simulink model "ThdRwRtStBkReclnIsPosChk"  (R2018b)
settings: Solver=FixedStepDiscrete  StartTime=0.0  StopTime=10.0  FixedStep=0.01  RelTol=1e-3
undefined symbols (not defined in the file or in its folder): KeSMSuThrdRwStBackPosDelta_Val, KeSMSuThrdRwStBackPosTolr_Val, KeSMSuVehicleModelConfig_Val
libraries: StIsPosChkLib x12, simulink x5
settings Model: Creator=sn2xws  LastModifiedBy=sn55gm
settings Model: ModifiedHistory=|
  | 2024.3.14
  | V2.3.0
  | Bug 813950 童锁Lock，Mode1_Easy Entry Mode 不应调用失败
  | 2024.6.25
  | V3.0.0 557模式流程
  | 2024.9.6 V3.0.1 新增Md56
  | 2024.10.14 V3.0.2 新增Md57，Md58
  | 2024.11.11 V3.0.3 vip模式到位置不看三排
  | 2024.11.27.V3.0.4 Md57 Md58接线遗漏
  | 2025.2.19 V3.8.0 Bug 991386 Md1 三排占座时未移动且报了成功
  | 25.7.1 V3.13.0 新增MD61 MD62
settings DataIOCC: SaveFormat=StructureWithTime
settings OptimizationCC: DefaultParameterBehavior=Inlined  EnhancedBackFolding=on  PassReuseOutputArgsAs=Individual arguments  ZeroExternalMemoryAtStartup=off  ZeroInternalMemoryAtStartup=off  OptimizeBlockOrder=speed  DifferentSizesBufferReuse=on  OptimizationCustomize=off
settings DebuggingCC: ParameterTunabilityLossMsg=error
settings ModelReferenceCC: ModelReferenceNumInstancesAllowed=Single
settings SFSimCC: MATLABDynamicMemAlloc=off
settings RTWCC: SystemTargetFile=autosar.tlc  GenCodeOnly=on  TemplateMakefile=ert_default_tmf  Description=AUTOSAR  GenerateReport=on  IncludeHyperlinkInReport=on  LaunchReport=on  GenerateTraceInfo=on  GenerateTraceReport=on  GenerateTraceReportSl=on  GenerateTraceReportSf=on  GenerateTraceReportEml=on
settings CodeAppCC: ForceParamTrailComments=on  IgnoreCustomStorageClasses=off  OperatorAnnotations=on  SimulinkDataObjDesc=on  SFDataObjDesc=on  InsertBlockDesc=on
settings STFCustomTargetCC: TargetLangStandard=C99 (ISO)  MultiwordLength=256  ParMdlRefBuildCompliant=on  CompOptLevelCompliant=on  IncludeMdlTerminateFcn=off  CombineOutputUpdateFcns=on  SuppressErrorStatus=on  ERTCustomFileBanners=on  SupportNonFinite=off  SupportComplex=off  SupportContinuousTime=off  SupportNonInlinedSFcns=off  RemoveResetFunc=on  MATLABClassNameForMDSCustomization=Simulink.SoftwareTarget.ERTCustomization  AutosarCompliant=on  UseToolchainInfoCompliant=on  LookupTableObjectStructAxisOrder=2,1,3,4,...  LUTObjectStructOrderEvenSpacing=Size,Table,Breakpoints  SystemTargetFile=autosar.tlc
settings ERTTargetCC: TargetLangStandard=C99 (ISO)  ConcurrentExecutionCompliant=off  IncludeMdlTerminateFcn=off  SuppressErrorStatus=on  SupportNonFinite=off  SupportComplex=off  ModelStepFunctionPrototypeControlCompliant=off  CPPClassGenCompliant=off  AutosarCompliant=on  LookupTableObjectStructAxisOrder=2,1,3,4,...  LUTObjectStructOrderEvenSpacing=Size,Table,Breakpoints  InlinedParameterPlacement=NonHierarchical  ERTCustomFileTemplate=example_file_process.tlc  ERTFilePackagingFormat=Compact

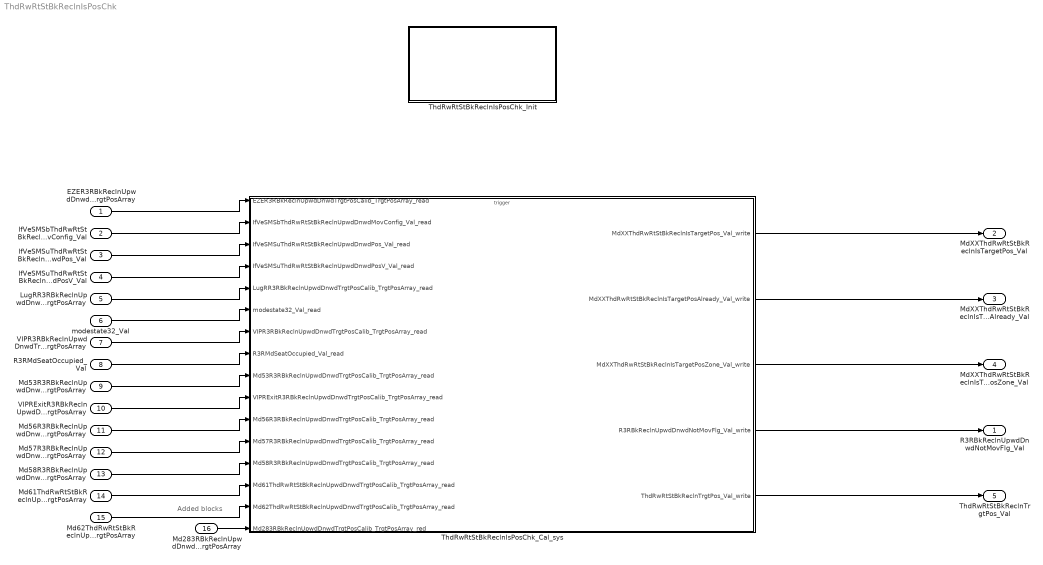
== system ThdRwRtStBkReclnIsPosChk ==
  note: Added blocks
  EZER3RBkReclnUpwdDnwdTrgtPosCalib_TrgtPosArray : Inport  Description=|  OutDataTypeStr=uint16  PortDimensions=3
      | 0:Pos
      | 1:Max
      | 2:Min
  IfVeSMSbThdRwRtStBkReclnUpwdDnwdMovConfig_Val : Inport  Port=2  OutDataTypeStr=boolean  PortDimensions=1
  IfVeSMSuThdRwRtStBkReclnUpwdDnwdPos_Val : Inport  Port=3  OutDataTypeStr=uint16  PortDimensions=1
  IfVeSMSuThdRwRtStBkReclnUpwdDnwdPosV_Val : Inport  Port=4  OutDataTypeStr=boolean  PortDimensions=1
  LugRR3RBkReclnUpwdDnwdTrgtPosCalib_TrgtPosArray : Inport  Description=|  Port=5  OutDataTypeStr=uint16  PortDimensions=3
      | 0:Pos
      | 1:Max
      | 2:Min
  modestate32_Val : Inport  Port=6  OutDataTypeStr=uint32  PortDimensions=1
  VIPR3RBkReclnUpwdDnwdTrgtPosCalib_TrgtPosArray : Inport  Description=|  Port=7  OutDataTypeStr=uint16  PortDimensions=3
      | 0:Pos
      | 1:Max
      | 2:Min
  R3RMdSeatOccupied_Val : Inport  Port=8  OutDataTypeStr=boolean  PortDimensions=1
  Md53R3RBkReclnUpwdDnwdTrgtPosCalib_TrgtPosArray : Inport  Description=|  Port=9  OutDataTypeStr=uint16  PortDimensions=3
      | 0:Pos
      | 1:Max
      | 2:Min
  VIPRExitR3RBkReclnUpwdDnwdTrgtPosCalib_TrgtPosArray : Inport  Description=|  Port=10  OutDataTypeStr=uint16  PortDimensions=3
      | 0:Pos
      | 1:Max
      | 2:Min
  Md56R3RBkReclnUpwdDnwdTrgtPosCalib_TrgtPosArray : Inport  Description=|  Port=11  OutDataTypeStr=uint16  PortDimensions=3
      | 0:Pos
      | 1:Max
      | 2:Min
  Md57R3RBkReclnUpwdDnwdTrgtPosCalib_TrgtPosArray : Inport  Description=|  Port=12  OutDataTypeStr=uint16  PortDimensions=3
      | 0:Pos
      | 1:Max
      | 2:Min
  Md58R3RBkReclnUpwdDnwdTrgtPosCalib_TrgtPosArray : Inport  Description=|  Port=13  OutDataTypeStr=uint16  PortDimensions=3
      | 0:Pos
      | 1:Max
      | 2:Min
  Md61ThdRwRtStBkReclnUpwdDnwdTrgtPosCalib_TrgtPosArray : Inport  Description=|  Port=14  OutDataTypeStr=uint16  PortDimensions=3
      | 0:Pos
      | 1:Max
      | 2:Min
  Md62ThdRwRtStBkReclnUpwdDnwdTrgtPosCalib_TrgtPosArray : Inport  Description=|  Port=15  OutDataTypeStr=uint16  PortDimensions=3
      | 0:Pos
      | 1:Max
      | 2:Min
  Md283RBkReclnUpwdDnwdTrgtPosCalib_TrgtPosArray : Inport  Description=|  Port=16  OutDataTypeStr=uint16  PortDimensions=3
      | 0:Pos
      | 1:Max
      | 2:Min
  ThdRwRtStBkReclnIsPosChk_Cal_sys : Subsystem
  ThdRwRtStBkReclnIsPosChk_Init : Subsystem
  R3RBkReclnUpwdDnwdNotMovFlg_Val : Outport  OutDataTypeStr=boolean  PortDimensions=1
  MdXXThdRwRtStBkReclnIsTargetPos_Val : Outport  Port=2  OutDataTypeStr=uint32  PortDimensions=1
  MdXXThdRwRtStBkReclnIsTargetPosAlready_Val : Outport  Port=3  OutDataTypeStr=uint32  PortDimensions=1
  MdXXThdRwRtStBkReclnIsTargetPosZone_Val : Outport  Port=4  OutDataTypeStr=uint32  PortDimensions=1
  ThdRwRtStBkReclnTrgtPos_Val : Outport  Port=5  OutDataTypeStr=uint16  PortDimensions=1
  wires:
  EZER3RBkReclnUpwdDnwdTrgtPosCalib_TrgtPosArray/1 -> ThdRwRtStBkReclnIsPosChk_Cal_sys/1(EZER3RBkReclnUpwdDnwdTrgtPosCalib_TrgtPosArray_read)
  IfVeSMSbThdRwRtStBkReclnUpwdDnwdMovConfig_Val/1 -> ThdRwRtStBkReclnIsPosChk_Cal_sys/2(IfVeSMSbThdRwRtStBkReclnUpwdDnwdMovConfig_Val_read)
  IfVeSMSuThdRwRtStBkReclnUpwdDnwdPos_Val/1 -> ThdRwRtStBkReclnIsPosChk_Cal_sys/3(IfVeSMSuThdRwRtStBkReclnUpwdDnwdPos_Val_read)
  IfVeSMSuThdRwRtStBkReclnUpwdDnwdPosV_Val/1 -> ThdRwRtStBkReclnIsPosChk_Cal_sys/4(IfVeSMSuThdRwRtStBkReclnUpwdDnwdPosV_Val_read)
  LugRR3RBkReclnUpwdDnwdTrgtPosCalib_TrgtPosArray/1 -> ThdRwRtStBkReclnIsPosChk_Cal_sys/5(LugRR3RBkReclnUpwdDnwdTrgtPosCalib_TrgtPosArray_read)
  modestate32_Val/1 -> ThdRwRtStBkReclnIsPosChk_Cal_sys/6(modestate32_Val_read)
  VIPR3RBkReclnUpwdDnwdTrgtPosCalib_TrgtPosArray/1 -> ThdRwRtStBkReclnIsPosChk_Cal_sys/7(VIPR3RBkReclnUpwdDnwdTrgtPosCalib_TrgtPosArray_read)
  ThdRwRtStBkReclnIsPosChk_Cal_sys/1(MdXXThdRwRtStBkReclnIsTargetPos_Val_write) -> MdXXThdRwRtStBkReclnIsTargetPos_Val/1
  ThdRwRtStBkReclnIsPosChk_Cal_sys/2(MdXXThdRwRtStBkReclnIsTargetPosAlready_Val_write) -> MdXXThdRwRtStBkReclnIsTargetPosAlready_Val/1
  ThdRwRtStBkReclnIsPosChk_Cal_sys/3(MdXXThdRwRtStBkReclnIsTargetPosZone_Val_write) -> MdXXThdRwRtStBkReclnIsTargetPosZone_Val/1
  ThdRwRtStBkReclnIsPosChk_Cal_sys/4(R3RBkReclnUpwdDnwdNotMovFlg_Val_write) -> R3RBkReclnUpwdDnwdNotMovFlg_Val/1
  ThdRwRtStBkReclnIsPosChk_Cal_sys/5(ThdRwRtStBkReclnTrgtPos_Val_write) -> ThdRwRtStBkReclnTrgtPos_Val/1
  R3RMdSeatOccupied_Val/1 -> ThdRwRtStBkReclnIsPosChk_Cal_sys/8(R3RMdSeatOccupied_Val_read)
  Md53R3RBkReclnUpwdDnwdTrgtPosCalib_TrgtPosArray/1 -> ThdRwRtStBkReclnIsPosChk_Cal_sys/9(Md53R3RBkReclnUpwdDnwdTrgtPosCalib_TrgtPosArray_read)
  VIPRExitR3RBkReclnUpwdDnwdTrgtPosCalib_TrgtPosArray/1 -> ThdRwRtStBkReclnIsPosChk_Cal_sys/10(VIPRExitR3RBkReclnUpwdDnwdTrgtPosCalib_TrgtPosArray_read)
  Md56R3RBkReclnUpwdDnwdTrgtPosCalib_TrgtPosArray/1 -> ThdRwRtStBkReclnIsPosChk_Cal_sys/11(Md56R3RBkReclnUpwdDnwdTrgtPosCalib_TrgtPosArray_read)
  Md57R3RBkReclnUpwdDnwdTrgtPosCalib_TrgtPosArray/1 -> ThdRwRtStBkReclnIsPosChk_Cal_sys/12(Md57R3RBkReclnUpwdDnwdTrgtPosCalib_TrgtPosArray_read)
  Md58R3RBkReclnUpwdDnwdTrgtPosCalib_TrgtPosArray/1 -> ThdRwRtStBkReclnIsPosChk_Cal_sys/13(Md58R3RBkReclnUpwdDnwdTrgtPosCalib_TrgtPosArray_read)
  Md61ThdRwRtStBkReclnUpwdDnwdTrgtPosCalib_TrgtPosArray/1 -> ThdRwRtStBkReclnIsPosChk_Cal_sys/14(Md61ThdRwRtStBkReclnUpwdDnwdTrgtPosCalib_TrgtPosArray_read)
  Md62ThdRwRtStBkReclnUpwdDnwdTrgtPosCalib_TrgtPosArray/1 -> ThdRwRtStBkReclnIsPosChk_Cal_sys/15(Md62ThdRwRtStBkReclnUpwdDnwdTrgtPosCalib_TrgtPosArray_read)
  Md283RBkReclnUpwdDnwdTrgtPosCalib_TrgtPosArray/1 -> ThdRwRtStBkReclnIsPosChk_Cal_sys/16(Md283RBkReclnUpwdDnwdTrgtPosCalib_TrgtPosArray_red)

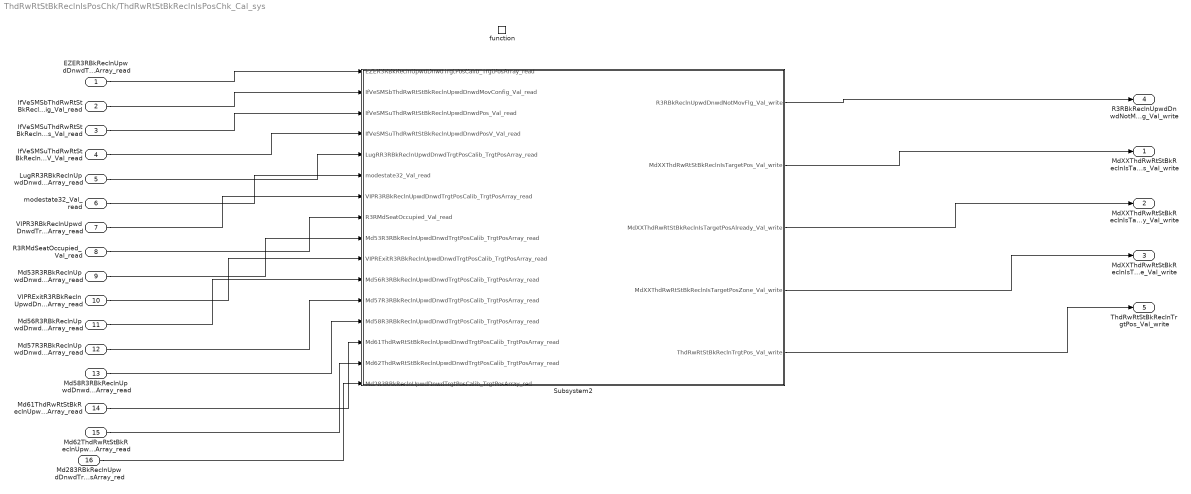
== system ThdRwRtStBkReclnIsPosChk/ThdRwRtStBkReclnIsPosChk_Cal_sys ==
  EZER3RBkReclnUpwdDnwdTrgtPosCalib_TrgtPosArray_read : Inport
  IfVeSMSbThdRwRtStBkReclnUpwdDnwdMovConfig_Val_read : Inport  Port=2
  IfVeSMSuThdRwRtStBkReclnUpwdDnwdPos_Val_read : Inport  Port=3
  IfVeSMSuThdRwRtStBkReclnUpwdDnwdPosV_Val_read : Inport  Port=4
  LugRR3RBkReclnUpwdDnwdTrgtPosCalib_TrgtPosArray_read : Inport  Port=5
  modestate32_Val_read : Inport  Port=6
  VIPR3RBkReclnUpwdDnwdTrgtPosCalib_TrgtPosArray_read : Inport  Port=7
  R3RMdSeatOccupied_Val_read : Inport  Port=8
  Md53R3RBkReclnUpwdDnwdTrgtPosCalib_TrgtPosArray_read : Inport  Port=9
  VIPRExitR3RBkReclnUpwdDnwdTrgtPosCalib_TrgtPosArray_read : Inport  Port=10
  Md56R3RBkReclnUpwdDnwdTrgtPosCalib_TrgtPosArray_read : Inport  Port=11
  Md57R3RBkReclnUpwdDnwdTrgtPosCalib_TrgtPosArray_read : Inport  Port=12
  Md58R3RBkReclnUpwdDnwdTrgtPosCalib_TrgtPosArray_read : Inport  Port=13
  Md61ThdRwRtStBkReclnUpwdDnwdTrgtPosCalib_TrgtPosArray_read : Inport  Port=14
  Md62ThdRwRtStBkReclnUpwdDnwdTrgtPosCalib_TrgtPosArray_read : Inport  Port=15
  Md283RBkReclnUpwdDnwdTrgtPosCalib_TrgtPosArray_red : Inport  Port=16
  function : TriggerPort  TriggerType=function-call  IsSimulinkFunction=on  FunctionName=ThdRwRtStBkReclnIsPosChk_Cal  VariantControl=(inherit)
  Subsystem2 : Subsystem
  MdXXThdRwRtStBkReclnIsTargetPos_Val_write : Outport
      settings: EnsureOutportIsVirtual=on
  MdXXThdRwRtStBkReclnIsTargetPosAlready_Val_write : Outport  Port=2
      settings: EnsureOutportIsVirtual=on
  MdXXThdRwRtStBkReclnIsTargetPosZone_Val_write : Outport  Port=3
      settings: EnsureOutportIsVirtual=on
  R3RBkReclnUpwdDnwdNotMovFlg_Val_write : Outport  Port=4
      settings: EnsureOutportIsVirtual=on
  ThdRwRtStBkReclnTrgtPos_Val_write : Outport  Port=5
      settings: EnsureOutportIsVirtual=on
  wires:
  Subsystem2/1(R3RBkReclnUpwdDnwdNotMovFlg_Val_write) -> R3RBkReclnUpwdDnwdNotMovFlg_Val_write/1
  Subsystem2/2(MdXXThdRwRtStBkReclnIsTargetPos_Val_write) -> MdXXThdRwRtStBkReclnIsTargetPos_Val_write/1
  Subsystem2/3(MdXXThdRwRtStBkReclnIsTargetPosAlready_Val_write) -> MdXXThdRwRtStBkReclnIsTargetPosAlready_Val_write/1
  Subsystem2/5(ThdRwRtStBkReclnTrgtPos_Val_write) -> ThdRwRtStBkReclnTrgtPos_Val_write/1
  Subsystem2/4(MdXXThdRwRtStBkReclnIsTargetPosZone_Val_write) -> MdXXThdRwRtStBkReclnIsTargetPosZone_Val_write/1
  EZER3RBkReclnUpwdDnwdTrgtPosCalib_TrgtPosArray_read/1 -> Subsystem2/1(EZER3RBkReclnUpwdDnwdTrgtPosCalib_TrgtPosArray_read)
  IfVeSMSbThdRwRtStBkReclnUpwdDnwdMovConfig_Val_read/1 -> Subsystem2/2(IfVeSMSbThdRwRtStBkReclnUpwdDnwdMovConfig_Val_read)
  IfVeSMSuThdRwRtStBkReclnUpwdDnwdPos_Val_read/1 -> Subsystem2/3(IfVeSMSuThdRwRtStBkReclnUpwdDnwdPos_Val_read)
  IfVeSMSuThdRwRtStBkReclnUpwdDnwdPosV_Val_read/1 -> Subsystem2/4(IfVeSMSuThdRwRtStBkReclnUpwdDnwdPosV_Val_read)
  LugRR3RBkReclnUpwdDnwdTrgtPosCalib_TrgtPosArray_read/1 -> Subsystem2/5(LugRR3RBkReclnUpwdDnwdTrgtPosCalib_TrgtPosArray_read)
  modestate32_Val_read/1 -> Subsystem2/6(modestate32_Val_read)
  VIPR3RBkReclnUpwdDnwdTrgtPosCalib_TrgtPosArray_read/1 -> Subsystem2/7(VIPR3RBkReclnUpwdDnwdTrgtPosCalib_TrgtPosArray_read)
  R3RMdSeatOccupied_Val_read/1 -> Subsystem2/8(R3RMdSeatOccupied_Val_read)
  Md53R3RBkReclnUpwdDnwdTrgtPosCalib_TrgtPosArray_read/1 -> Subsystem2/9(Md53R3RBkReclnUpwdDnwdTrgtPosCalib_TrgtPosArray_read)
  VIPRExitR3RBkReclnUpwdDnwdTrgtPosCalib_TrgtPosArray_read/1 -> Subsystem2/10(VIPRExitR3RBkReclnUpwdDnwdTrgtPosCalib_TrgtPosArray_read)
  Md56R3RBkReclnUpwdDnwdTrgtPosCalib_TrgtPosArray_read/1 -> Subsystem2/11(Md56R3RBkReclnUpwdDnwdTrgtPosCalib_TrgtPosArray_read)
  Md57R3RBkReclnUpwdDnwdTrgtPosCalib_TrgtPosArray_read/1 -> Subsystem2/12(Md57R3RBkReclnUpwdDnwdTrgtPosCalib_TrgtPosArray_read)
  Md58R3RBkReclnUpwdDnwdTrgtPosCalib_TrgtPosArray_read/1 -> Subsystem2/13(Md58R3RBkReclnUpwdDnwdTrgtPosCalib_TrgtPosArray_read)
  Md61ThdRwRtStBkReclnUpwdDnwdTrgtPosCalib_TrgtPosArray_read/1 -> Subsystem2/14(Md61ThdRwRtStBkReclnUpwdDnwdTrgtPosCalib_TrgtPosArray_read)
  Md62ThdRwRtStBkReclnUpwdDnwdTrgtPosCalib_TrgtPosArray_read/1 -> Subsystem2/15(Md62ThdRwRtStBkReclnUpwdDnwdTrgtPosCalib_TrgtPosArray_read)
  Md283RBkReclnUpwdDnwdTrgtPosCalib_TrgtPosArray_red/1 -> Subsystem2/16(Md283RBkReclnUpwdDnwdTrgtPosCalib_TrgtPosArray_red)

== system ThdRwRtStBkReclnIsPosChk/ThdRwRtStBkReclnIsPosChk_Init ==
  note: Added blocks
  note: Added blocks
  note: Added blocks
  Event Listener : EventListener  EventName=reset
  PA_KeSMSuThrdRwStBackPosDelta_Val : Constant  Value=KeSMSuThrdRwStBackPosDelta_Val
  PA_KeSMSuThrdRwStBackPosTolr_Val : Constant  Value=KeSMSuThrdRwStBackPosTolr_Val
  PA_KeSMSuVehicleModelConfig_Val : Constant  Value=KeSMSuVehicleModelConfig_Val
  Terminator_1 : Terminator
  Terminator_2 : Terminator
  Terminator_3 : Terminator
  wires:
  PA_KeSMSuThrdRwStBackPosDelta_Val/1 -> Terminator_1/1
  PA_KeSMSuThrdRwStBackPosTolr_Val/1 -> Terminator_2/1
  PA_KeSMSuVehicleModelConfig_Val/1 -> Terminator_3/1

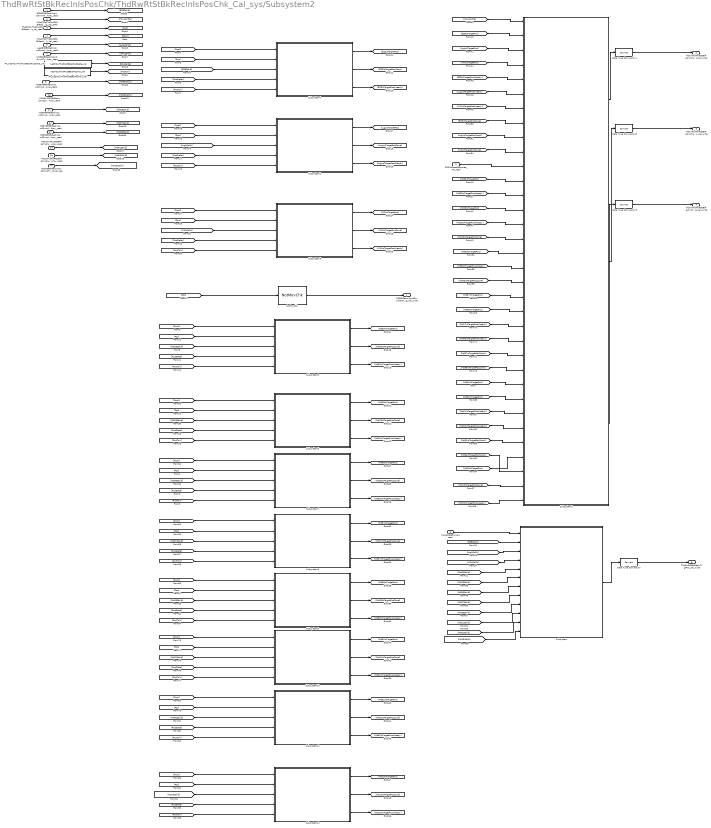
== system ThdRwRtStBkReclnIsPosChk/ThdRwRtStBkReclnIsPosChk_Cal_sys/Subsystem2 ==
  EZER3RBkReclnUpwdDnwdTrgtPosCalib_TrgtPosArray_read : Inport
  IfVeSMSbThdRwRtStBkReclnUpwdDnwdMovConfig_Val_read : Inport  Port=2
  IfVeSMSuThdRwRtStBkReclnUpwdDnwdPos_Val_read : Inport  Port=3
  IfVeSMSuThdRwRtStBkReclnUpwdDnwdPosV_Val_read : Inport  Port=4
  LugRR3RBkReclnUpwdDnwdTrgtPosCalib_TrgtPosArray_read : Inport  Port=5
  modestate32_Val_read : Inport  Port=6
  VIPR3RBkReclnUpwdDnwdTrgtPosCalib_TrgtPosArray_read : Inport  Port=7
  R3RMdSeatOccupied_Val_read : Inport  Port=8
  Md53R3RBkReclnUpwdDnwdTrgtPosCalib_TrgtPosArray_read : Inport  Port=9
  VIPRExitR3RBkReclnUpwdDnwdTrgtPosCalib_TrgtPosArray_read : Inport  Port=10
  Md56R3RBkReclnUpwdDnwdTrgtPosCalib_TrgtPosArray_read : Inport  Port=11
  Md57R3RBkReclnUpwdDnwdTrgtPosCalib_TrgtPosArray_read : Inport  Port=12
  Md58R3RBkReclnUpwdDnwdTrgtPosCalib_TrgtPosArray_read : Inport  Port=13
  Md61ThdRwRtStBkReclnUpwdDnwdTrgtPosCalib_TrgtPosArray_read : Inport  Port=14
  Md62ThdRwRtStBkReclnUpwdDnwdTrgtPosCalib_TrgtPosArray_read : Inport  Port=15
  Md283RBkReclnUpwdDnwdTrgtPosCalib_TrgtPosArray_red : Inport  Port=16
  Data Type Conversion{,1..3} (4 alike) : DataTypeConversion
  NotMovChk : StIsPosChkLib/NotMovChk  SystemSampleTime=-1
  PA_KeSMSuThrdRwStBackPosDelta_Val : Constant  Value=KeSMSuThrdRwStBackPosDelta_Val
  PA_KeSMSuThrdRwStBackPosTolr_Val : Constant  Value=KeSMSuThrdRwStBackPosTolr_Val
  Subsystem : Subsystem
  Subsystem1 : Subsystem
  Subsystem10 : Subsystem
  Subsystem11 : Subsystem
  Subsystem12 : Subsystem
  Subsystem2 : Subsystem
  Subsystem3 : Subsystem
  Subsystem4 : Subsystem
  Subsystem5 : Subsystem
  Subsystem6 : Subsystem
  Subsystem7 : Subsystem
  Subsystem8 : Subsystem
  Subsystem9 : Subsystem
  R3RBkReclnUpwdDnwdNotMovFlg_Val_write : Outport
      settings: EnsureOutportIsVirtual=on
  MdXXThdRwRtStBkReclnIsTargetPos_Val_write : Outport  Port=2
      settings: EnsureOutportIsVirtual=on
  MdXXThdRwRtStBkReclnIsTargetPosAlready_Val_write : Outport  Port=3
      settings: EnsureOutportIsVirtual=on
  MdXXThdRwRtStBkReclnIsTargetPosZone_Val_write : Outport  Port=4
      settings: EnsureOutportIsVirtual=on
  ThdRwRtStBkReclnTrgtPos_Val_write : Outport  Port=5
      settings: EnsureOutportIsVirtual=on
  wires:
  Data Type Conversion3/1 -> MdXXThdRwRtStBkReclnIsTargetPosZone_Val_write/1
  Data Type Conversion2/1 -> MdXXThdRwRtStBkReclnIsTargetPosAlready_Val_write/1
  [LugLIsTargetPos] -> Subsystem1/3(LugLIsTargetPos)
  [EZECalib] -> Subsystem4/3(CalibArray)
  [Pos] -> Subsystem3/2(Pos)
  Subsystem4/1(IsPos) -> [EZEIsTargetPos]
  [PosDelta] -> Subsystem2/4(Delta)
  IfVeSMSuThdRwRtStBkReclnUpwdDnwdPosV_Val_read/1 -> [PosV]
  Subsystem3/1(IsPos) -> [VIPLIsTargetPos]
  Subsystem3/2(IsPosZone) -> [VIPLIsTargetPosZone]
  [PosV] -> Subsystem2/1(PosV)
  [LugLIsTargetPosAlready] -> Subsystem1/6(LugLIsTargetPosAlready)
  [PosV] -> Subsystem4/1(PosV)
  VIPR3RBkReclnUpwdDnwdTrgtPosCalib_TrgtPosArray_read/1 -> [VIPLCalib]
  IfVeSMSbThdRwRtStBkReclnUpwdDnwdMovConfig_Val_read/1 -> [MovConfig]
  Subsystem2/2(IsPosZone) -> [LugLIsTargetPosZone]
  [VIPLCalib] -> Subsystem3/3(CalibArray)
  [Pos] -> Subsystem2/2(Pos)
  LugRR3RBkReclnUpwdDnwdTrgtPosCalib_TrgtPosArray_read/1 -> [LugLCalib]
  [PosV] -> Subsystem3/1(PosV)
  [EZEIsTargetPos] -> Subsystem1/2(EZEIsTargetPos)
  [PosTolr] -> Subsystem4/5(Tolr)
  [Pos] -> Subsystem4/2(Pos)
  [VIPLIsTargetPosAlready] -> Subsystem1/7(VIPLIsTargetPosAlready)
  [VIPLCalib] -> Subsystem/4(VIPLCalib)
  PA_KeSMSuThrdRwStBackPosTolr_Val/1 -> [PosTolr]
  [VIPLIsTargetPos] -> Subsystem1/4(VIPLIsTargetPos)
  Subsystem1/2(IsTargetPosAlready) -> Data Type Conversion2/1
  Data Type Conversion1/1 -> MdXXThdRwRtStBkReclnIsTargetPos_Val_write/1
  [Pos] -> NotMovChk/1
  [LugLCalib] -> Subsystem/3(EZQCalib)
  [EZEIsTargetPosAlready] -> Subsystem1/5(EZEIsTargetPosAlready)
  [LugLIsTargetPosZone] -> Subsystem1/9(LugLIsTargetPosZone)
  [EZEIsTargetPosZone] -> Subsystem1/8(EZEIsTargetPosZone)
  Subsystem1/3(IsTargetPosZone) -> Data Type Conversion3/1
  Subsystem1/1(IsTargetPos) -> Data Type Conversion1/1
  EZER3RBkReclnUpwdDnwdTrgtPosCalib_TrgtPosArray_read/1 -> [EZECalib]
  [MovConfig] -> Subsystem1/1(MovConfig)
  Subsystem4/3(IsPosAlready) -> [EZEIsTargetPosAlready]
  Subsystem4/2(IsPosZone) -> [EZEIsTargetPosZone]
  Subsystem2/1(IsPos) -> [LugLIsTargetPos]
  modestate32_Val_read/1 -> Subsystem/1(modestate32_Val_read)
  IfVeSMSuThdRwRtStBkReclnUpwdDnwdPos_Val_read/1 -> [Pos]
  [PosTolr] -> Subsystem3/5(Tolr)
  Subsystem2/3(IsPosAlready) -> [LugLIsTargetPosAlready]
  Subsystem/1(TrgtPos) -> Data Type Conversion/1
  PA_KeSMSuThrdRwStBackPosDelta_Val/1 -> [PosDelta]
  Data Type Conversion/1 -> ThdRwRtStBkReclnTrgtPos_Val_write/1
  NotMovChk/1 -> R3RBkReclnUpwdDnwdNotMovFlg_Val_write/1
  [LugLCalib] -> Subsystem2/3(CalibArray)
  [PosTolr] -> Subsystem2/5(Tolr)
  [PosDelta] -> Subsystem4/4(Delta)
  Subsystem3/3(IsPosAlready) -> [VIPLIsTargetPosAlready]
  [PosDelta] -> Subsystem3/4(Delta)
  [EZECalib] -> Subsystem/2(EZECalib)
  [VIPLIsTargetPosZone] -> Subsystem1/10(VIPLIsTargetPosZone)
  R3RMdSeatOccupied_Val_read/1 -> Subsystem1/11(R3RMdSeatOccupied_Val_read)
  Md53R3RBkReclnUpwdDnwdTrgtPosCalib_TrgtPosArray_read/1 -> [Md53Calib]
  [Md53Calib] -> Subsystem5/3(CalibArray)
  [PosV] -> Subsystem5/1(PosV)
  [Pos] -> Subsystem5/2(Pos)
  [PosDelta] -> Subsystem5/4(Delta)
  [PosTolr] -> Subsystem5/5(Tolr)
  Subsystem5/3(IsPosAlready) -> [Md53IsTargetPosAlready]
  Subsystem5/2(IsPosZone) -> [Md53IsTargetPosZone]
  Subsystem5/1(IsPos) -> [Md53IsTargetPos]
  [Md53Calib] -> Subsystem/5(Md53Calib)
  [Md53IsTargetPos] -> Subsystem1/12(Md53IsTargetPos)
  [Md53IsTargetPosAlready] -> Subsystem1/13(Md53IsTargetPosAlready)
  Subsystem6/1(IsPos) -> [Md28IsTargetPos]
  Subsystem6/2(IsPosZone) -> [Md28IsTargetPosZone]
  Subsystem6/3(IsPosAlready) -> [Md28IsTargetPosAlready]
  [PosTolr] -> Subsystem6/5(Tolr)
  [PosDelta] -> Subsystem6/4(Delta)
  [Pos] -> Subsystem6/2(Pos)
  [PosV] -> Subsystem6/1(PosV)
  [Md28Calib] -> Subsystem6/3(CalibArray)
  [Md28Calib] -> Subsystem/6(Md28Calib)
  [Md28IsTargetPos] -> Subsystem1/14(Md28IsTargetPos)
  [Md28IsTargetPosZone] -> Subsystem1/16(Md28IsTargetPosZone)
  [Md28IsTargetPosAlready] -> Subsystem1/15(Md28IsTargetPosAlready)
  Md56R3RBkReclnUpwdDnwdTrgtPosCalib_TrgtPosArray_read/1 -> [Md56Calib]
  [Md56Calib] -> Subsystem7/3(CalibArray)
  [PosV] -> Subsystem7/1(PosV)
  [Pos] -> Subsystem7/2(Pos)
  [PosDelta] -> Subsystem7/4(Delta)
  [PosTolr] -> Subsystem7/5(Tolr)
  Subsystem7/3(IsPosAlready) -> [Md56IsTargetPosAlready]
  Subsystem7/2(IsPosZone) -> [Md56IsTargetPosZone]
  Subsystem7/1(IsPos) -> [Md56IsTargetPos]
  [Md56Calib] -> Subsystem/7(Md56Calib)
  [Md56IsTargetPosAlready] -> Subsystem1/18(Md56IsTargetPosAlready)
  [Md56IsTargetPosZone] -> Subsystem1/19(Md56IsTargetPosZone)
  [Md56IsTargetPos] -> Subsystem1/17(Md56IsTargetPos)
  Md58R3RBkReclnUpwdDnwdTrgtPosCalib_TrgtPosArray_read/1 -> [Md58Calib]
  Md57R3RBkReclnUpwdDnwdTrgtPosCalib_TrgtPosArray_read/1 -> [Md57Calib]
  Subsystem8/1(IsPos) -> [Md57IsTargetPos]
  Subsystem8/2(IsPosZone) -> [Md57IsTargetPosZone]
  Subsystem8/3(IsPosAlready) -> [Md57IsTargetPosAlready]
  [PosTolr] -> Subsystem8/5(Tolr)
  [PosDelta] -> Subsystem8/4(Delta)
  [Pos] -> Subsystem8/2(Pos)
  [PosV] -> Subsystem8/1(PosV)
  [Md57Calib] -> Subsystem8/3(CalibArray)
  [Md58Calib] -> Subsystem9/3(CalibArray)
  [PosV] -> Subsystem9/1(PosV)
  [Pos] -> Subsystem9/2(Pos)
  [PosDelta] -> Subsystem9/4(Delta)
  [PosTolr] -> Subsystem9/5(Tolr)
  Subsystem9/3(IsPosAlready) -> [Md58IsTargetPosAlready]
  Subsystem9/2(IsPosZone) -> [Md58IsTargetPosZone]
  Subsystem9/1(IsPos) -> [Md58IsTargetPos]
  [Md58Calib] -> Subsystem/9(Md58Calib)
  [Md57Calib] -> Subsystem/8(Md57Calib)
  [Md58IsTargetPos] -> Subsystem1/21(Md58IsTargetPos)
  [Md57IsTargetPos] -> Subsystem1/20(Md57IsTargetPos)
  [Md57IsTargetPosAlready] -> Subsystem1/22(Md57IsTargetPosAlready)
  [Md58IsTargetPosAlready] -> Subsystem1/23(Md58IsTargetPosAlready)
  [Md57IsTargetPosZone] -> Subsystem1/24(Md57IsTargetPosZone)
  [Md58IsTargetPosZone] -> Subsystem1/25(Md58IsTargetPosZone)
  Md61ThdRwRtStBkReclnUpwdDnwdTrgtPosCalib_TrgtPosArray_read/1 -> [Md61Calib]
  Md62ThdRwRtStBkReclnUpwdDnwdTrgtPosCalib_TrgtPosArray_read/1 -> [Md62Calib]
  Subsystem10/1(IsPos) -> [Md61IsTargetPos]
  Subsystem10/2(IsPosZone) -> [Md61IsTargetPosZone]
  Subsystem10/3(IsPosAlready) -> [Md61IsTargetPosAlready]
  [PosTolr] -> Subsystem10/5(Tolr)
  [PosDelta] -> Subsystem10/4(Delta)
  [Pos] -> Subsystem10/2(Pos)
  [PosV] -> Subsystem10/1(PosV)
  [Md61Calib] -> Subsystem10/3(CalibArray)
  [Md62Calib] -> Subsystem11/3(CalibArray)
  [PosV] -> Subsystem11/1(PosV)
  [Pos] -> Subsystem11/2(Pos)
  [PosDelta] -> Subsystem11/4(Delta)
  [PosTolr] -> Subsystem11/5(Tolr)
  Subsystem11/3(IsPosAlready) -> [Md62IsTargetPosAlready]
  Subsystem11/2(IsPosZone) -> [Md62IsTargetPosZone]
  Subsystem11/1(IsPos) -> [Md62IsTargetPos]
  [Md61Calib] -> Subsystem/10(Md61Calib)
  [Md62Calib] -> Subsystem/11(Md62Calib)
  [Md61IsTargetPos] -> Subsystem1/26(Md61IsTargetPos)
  [Md62IsTargetPosZone] -> Subsystem1/32(Md62IsTargetPosZone)
  [Md61IsTargetPosZone] -> Subsystem1/30(Md61IsTargetPosZone)
  [Md62IsTargetPosAlready] -> Subsystem1/29(Md62IsTargetPosAlready)
  [Md61IsTargetPosAlready] -> Subsystem1/28(Md61IsTargetPosAlready)
  [Md62IsTargetPos] -> Subsystem1/27(Md62IsTargetPos)
  VIPRExitR3RBkReclnUpwdDnwdTrgtPosCalib_TrgtPosArray_read/1 -> [Md28Calib]
  Md283RBkReclnUpwdDnwdTrgtPosCalib_TrgtPosArray_red/1 -> [Md15Calib]
  [PosV] -> Subsystem12/1(PosV)
  Subsystem12/2(IsPosZone) -> [Md15IsTargetPosZone]
  Subsystem12/1(IsPos) -> [Md15IsTargetPos]
  [PosTolr] -> Subsystem12/5(Tolr)
  [PosDelta] -> Subsystem12/4(Delta)
  [Md15Calib] -> Subsystem12/3(CalibArray)
  Subsystem12/3(IsPosAlready) -> [Md15IsTargetPosAlready]
  [Pos] -> Subsystem12/2(Pos)
  [Md15IsTargetPos] -> Subsystem1/31(Md15IsTargetPos)
  [Md15IsTargetPosZone] -> Subsystem1/33(Md15IsTargetPosZone)
  [Md15IsTargetPosAlready] -> Subsystem1/34(Md15IsTargetPosAlready)
  [Md15Calib] -> Subsystem/12(Md15Calib)

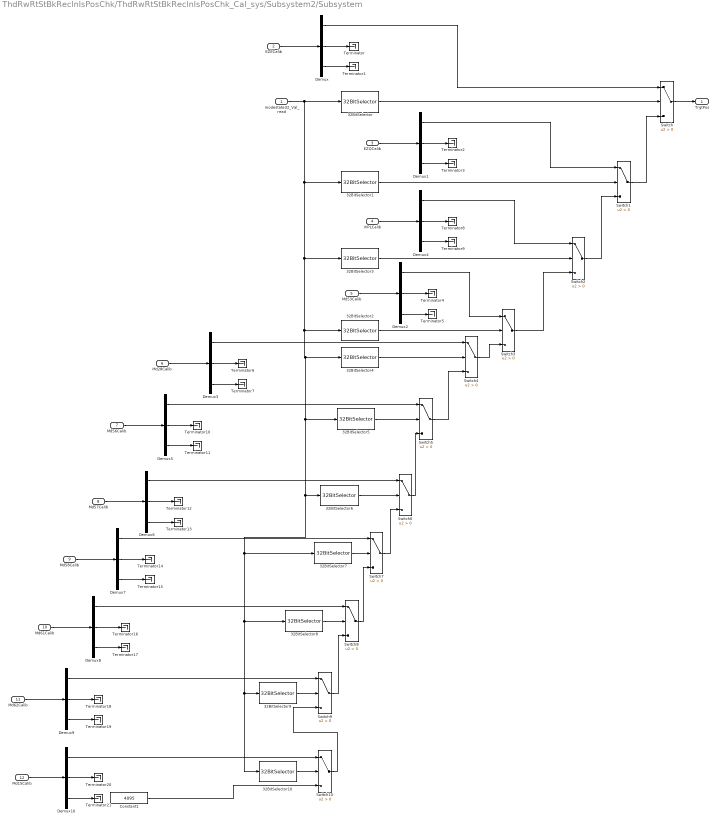
== system ThdRwRtStBkReclnIsPosChk/ThdRwRtStBkReclnIsPosChk_Cal_sys/Subsystem2/Subsystem ==
  modestate32_Val_read : Inport
  EZECalib : Inport  Port=2
  EZQCalib : Inport  Port=3
  VIPLCalib : Inport  Port=4
  Md53Calib : Inport  Port=5
  Md28Calib : Inport  Port=6
  Md56Calib : Inport  Port=7
  Md57Calib : Inport  Port=8
  Md58Calib : Inport  Port=9
  Md61Calib : Inport  Port=10
  Md62Calib : Inport  Port=11
  Md15Calib : Inport  Port=12
  32BitSelector : StIsPosChkLib/32BitSelector  BitNum=0
  32BitSelector1 : StIsPosChkLib/32BitSelector  BitNum=8
  32BitSelector10 : StIsPosChkLib/32BitSelector  BitNum=14
  32BitSelector2 : StIsPosChkLib/32BitSelector  BitNum=17
  32BitSelector3 : StIsPosChkLib/32BitSelector  BitNum=11
  32BitSelector4 : StIsPosChkLib/32BitSelector  BitNum=27
  32BitSelector5 : StIsPosChkLib/32BitSelector  BitNum=24
  32BitSelector6 : StIsPosChkLib/32BitSelector  BitNum=20
  32BitSelector7 : StIsPosChkLib/32BitSelector  BitNum=21
  32BitSelector8 : StIsPosChkLib/32BitSelector  BitNum=5
  32BitSelector9 : StIsPosChkLib/32BitSelector  BitNum=6
  Constant1 : Constant  Value=4095  OutDataTypeStr=uint16
  Demux{,1..10} (11 alike) : Demux  Outputs=3
  Switch{,1..10} (11 alike) : Switch  Criteria=u2 > Threshold
  Terminator{,1..21} (22 alike) : Terminator
  TrgtPos : Outport
      settings: EnsureOutportIsVirtual=on
  wires:
  32BitSelector/1 -> Switch/2
  Demux/1 -> Switch/1
  Demux/3 -> Terminator1/1
  Demux/2 -> Terminator/1
  EZECalib/1 -> Demux/1
  EZQCalib/1 -> Demux1/1
  Demux1/2 -> Terminator2/1
  Demux1/3 -> Terminator3/1
  Demux1/1 -> Switch1/1
  Switch/1 -> TrgtPos/1
  Switch1/1 -> Switch/3
  32BitSelector1/1 -> Switch1/2
  32BitSelector3/1 -> Switch2/2
  Demux4/3 -> Terminator9/1
  Demux4/2 -> Terminator8/1
  VIPLCalib/1 -> Demux4/1
  Switch2/1 -> Switch1/3
  Demux4/1 -> Switch2/1
  Switch3/1 -> Switch2/3
  32BitSelector2/1 -> Switch3/2
  Md53Calib/1 -> Demux2/1
  Demux2/2 -> Terminator4/1
  Demux2/3 -> Terminator5/1
  Demux2/1 -> Switch3/1
  Demux3/1 -> Switch4/1
  Demux3/3 -> Terminator7/1
  Demux3/2 -> Terminator6/1
  Md28Calib/1 -> Demux3/1
  Switch4/1 -> Switch3/3
  32BitSelector4/1 -> Switch4/2
  Switch5/1 -> Switch4/3
  32BitSelector5/1 -> Switch5/2
  Md56Calib/1 -> Demux5/1
  Demux5/2 -> Terminator10/1
  Demux5/3 -> Terminator11/1
  Demux5/1 -> Switch5/1
  Switch6/1 -> Switch5/3
  Switch7/1 -> Switch6/3
  32BitSelector6/1 -> Switch6/2
  32BitSelector7/1 -> Switch7/2
  Demux6/1 -> Switch6/1
  Demux6/3 -> Terminator13/1
  Demux6/2 -> Terminator12/1
  Md57Calib/1 -> Demux6/1
  Md58Calib/1 -> Demux7/1
  Demux7/2 -> Terminator14/1
  Demux7/3 -> Terminator15/1
  Demux7/1 -> Switch7/1
  Switch8/1 -> Switch7/3
  32BitSelector8/1 -> Switch8/2
  Switch9/1 -> Switch8/3
  32BitSelector9/1 -> Switch9/2
  Demux8/1 -> Switch8/1
  Demux8/3 -> Terminator17/1
  Demux8/2 -> Terminator16/1
  Md61Calib/1 -> Demux8/1
  Md62Calib/1 -> Demux9/1
  Demux9/2 -> Terminator18/1
  Demux9/3 -> Terminator19/1
  Demux9/1 -> Switch9/1
  Constant1/1 -> Switch10/3
  Md15Calib/1 -> Demux10/1
  Demux10/1 -> Switch10/1
  32BitSelector10/1 -> Switch10/2
  modestate32_Val_read/1 -> 32BitSelector7/1, 32BitSelector8/1, 32BitSelector10/1, 32BitSelector9/1, 32BitSelector6/1, 32BitSelector5/1, 32BitSelector4/1, 32BitSelector2/1, 32BitSelector3/1, 32BitSelector1/1, 32BitSelector/1
  Demux10/3 -> Terminator21/1
  Demux10/2 -> Terminator20/1
  Switch10/1 -> Switch9/3

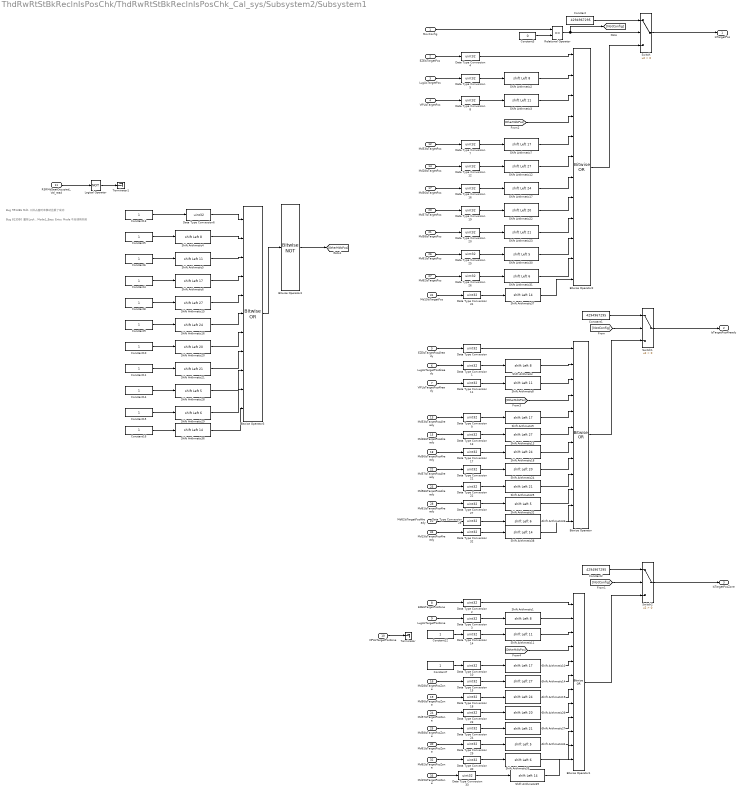
== system ThdRwRtStBkReclnIsPosChk/ThdRwRtStBkReclnIsPosChk_Cal_sys/Subsystem2/Subsystem1 ==
  note: Bug 991386 Md1 三排占座时未移动且报了成功
  note: Bug 813950 童锁Lock，Mode1_Easy Entry Mode 不应调用失败
  MovConfig : Inport
  EZEIsTargetPos : Inport  Port=2
  LugLIsTargetPos : Inport  Port=3
  VIPLIsTargetPos : Inport  Port=4
  EZEIsTargetPosAlready : Inport  Port=5
  LugLIsTargetPosAlready : Inport  Port=6
  VIPLIsTargetPosAlready : Inport  Port=7
  EZEIsTargetPosZone : Inport  Port=8
  LugLIsTargetPosZone : Inport  Port=9
  VIPLIsTargetPosZone : Inport  Port=10
  R3RMdSeatOccupied_Val_read : Inport  Port=11
  Md53IsTargetPos : Inport  Port=12
  Md53IsTargetPosAlready : Inport  Port=13
  Md28IsTargetPos : Inport  Port=14
  Md28IsTargetPosAlready : Inport  Port=15
  Md28IsTargetPosZone : Inport  Port=16
  Md56IsTargetPos : Inport  Port=17
  Md56IsTargetPosAlready : Inport  Port=18
  Md56IsTargetPosZone : Inport  Port=19
  Md57IsTargetPos : Inport  Port=20
  Md58IsTargetPos : Inport  Port=21
  Md57IsTargetPosAlready : Inport  Port=22
  Md58IsTargetPosAlready : Inport  Port=23
  Md57IsTargetPosZone : Inport  Port=24
  Md58IsTargetPosZone : Inport  Port=25
  Md61IsTargetPos : Inport  Port=26
  Md62IsTargetPos : Inport  Port=27
  Md61IsTargetPosAlready : Inport  Port=28
  Md62IsTargetPosAlready : Inport  Port=29
  Md61IsTargetPosZone : Inport  Port=30
  Md15IsTargetPos : Inport  Port=31
  Md62IsTargetPosZone : Inport  Port=32
  Md15IsTargetPosZone : Inport  Port=33
  Md15IsTargetPosAlready : Inport  Port=34
  Bitwise Operator : simulink/Logic and Bit Operations/Bitwise Operator  logicop=OR  UseBitMask=off  NumInputPorts=12  BitMask=bin2dec('11011001')  BitMaskRealWorld=Stored Integer
  Bitwise Operator1 : simulink/Logic and Bit Operations/Bitwise Operator  logicop=OR  UseBitMask=off  NumInputPorts=12  BitMask=bin2dec('11011001')  BitMaskRealWorld=Stored Integer
  Bitwise Operator2 : simulink/Logic and Bit Operations/Bitwise Operator  logicop=OR  UseBitMask=off  NumInputPorts=12  BitMask=bin2dec('11011001')  BitMaskRealWorld=Stored Integer
  Bitwise Operator3 : simulink/Logic and Bit Operations/Bitwise Operator  logicop=OR  UseBitMask=off  NumInputPorts=11  BitMask=bin2dec('11011001')  BitMaskRealWorld=Stored Integer
  Bitwise Operator4 : simulink/Logic and Bit Operations/Bitwise Operator  logicop=NOT  UseBitMask=off  BitMask=bin2dec('11011001')  BitMaskRealWorld=Stored Integer
  Constant : Constant  Value=4294967295  OutDataTypeStr=uint32
  Constant1 : Constant  Value=4294967295  OutDataTypeStr=uint32
  Constant{4..16} (13 alike) : Constant  OutDataTypeStr=uint32
  Constant2 : Constant  Value=4294967295  OutDataTypeStr=uint32
  Constant3 : Constant  Value=0  OutDataTypeStr=uint8
  Data Type Conversion{,1..33} (34 alike) : DataTypeConversion  OutDataTypeStr=uint32
  Logical Operator : Logic  Operator=NOT  AllPortsSameDT=off  OutDataTypeStr=boolean
  Relational Operator : RelationalOperator  Operator===  OutDataTypeStr=boolean  RndMeth=Simplest
  Shift Arithmetic{,1..2,4} (4 alike) : ArithShift  BitShiftNumber=8  BitShiftDirection=Left
  Shift Arithmetic{6..7,9..10} (4 alike) : ArithShift  BitShiftNumber=17  BitShiftDirection=Left
  Shift Arithmetic{3,5,8,11} (4 alike) : ArithShift  BitShiftNumber=11  BitShiftDirection=Left
  Shift Arithmetic{12..15} (4 alike) : ArithShift  BitShiftNumber=27  BitShiftDirection=Left
  Shift Arithmetic{16..19} (4 alike) : ArithShift  BitShiftNumber=24  BitShiftDirection=Left
  Shift Arithmetic{20,22,24,26} (4 alike) : ArithShift  BitShiftNumber=20  BitShiftDirection=Left
  Shift Arithmetic{21,23,25,27} (4 alike) : ArithShift  BitShiftNumber=21  BitShiftDirection=Left
  Shift Arithmetic{28,30,32,34} (4 alike) : ArithShift  BitShiftNumber=5  BitShiftDirection=Left
  Shift Arithmetic{29,31,33,35} (4 alike) : ArithShift  BitShiftNumber=6  BitShiftDirection=Left
  Shift Arithmetic{36..39} (4 alike) : ArithShift  BitShiftNumber=14  BitShiftDirection=Left
  Switch : Switch  Criteria=u2 > Threshold
  Switch1 : Switch  Criteria=u2 > Threshold
  Switch2 : Switch  Criteria=u2 > Threshold
  Terminator : Terminator
  Terminator1 : Terminator
  IsTargetPos : Outport
      settings: EnsureOutportIsVirtual=on
  IsTargetPosAlready : Outport  Port=2
      settings: EnsureOutportIsVirtual=on
  IsTargetPosZone : Outport  Port=3
      settings: EnsureOutportIsVirtual=on
  wires:
  Constant3/1 -> Relational Operator/2
  Constant/1 -> Switch/1
  Relational Operator/1 -> [NotConfig], Switch/2
  MovConfig/1 -> Relational Operator/1
  Switch/1 -> IsTargetPos/1
  [NotConfig] -> Switch1/2
  Constant1/1 -> Switch1/1
  Switch1/1 -> IsTargetPosAlready/1
  Switch2/1 -> IsTargetPosZone/1
  Constant2/1 -> Switch2/1
  [NotConfig] -> Switch2/2
  Data Type Conversion1/1 -> Shift Arithmetic/1
  Data Type Conversion/1 -> Bitwise Operator/1
  Shift Arithmetic/1 -> Bitwise Operator/2
  Shift Arithmetic1/1 -> Bitwise Operator1/2
  Data Type Conversion2/1 -> Bitwise Operator1/1
  Data Type Conversion3/1 -> Shift Arithmetic1/1
  Bitwise Operator1/1 -> Switch2/3
  Bitwise Operator/1 -> Switch1/3
  Shift Arithmetic2/1 -> Bitwise Operator2/2
  Data Type Conversion4/1 -> Bitwise Operator2/1
  Data Type Conversion5/1 -> Shift Arithmetic2/1
  Bitwise Operator2/1 -> Switch/3
  EZEIsTargetPos/1 -> Data Type Conversion4/1
  LugLIsTargetPos/1 -> Data Type Conversion5/1
  LugLIsTargetPosZone/1 -> Data Type Conversion3/1
  EZEIsTargetPosZone/1 -> Data Type Conversion2/1
  LugLIsTargetPosAlready/1 -> Data Type Conversion1/1
  EZEIsTargetPosAlready/1 -> Data Type Conversion/1
  Data Type Conversion8/1 -> Shift Arithmetic3/1
  VIPLIsTargetPos/1 -> Data Type Conversion8/1
  VIPLIsTargetPosAlready/1 -> Data Type Conversion11/1
  Data Type Conversion11/1 -> Shift Arithmetic8/1
  Shift Arithmetic8/1 -> Bitwise Operator/3
  Data Type Conversion14/1 -> Shift Arithmetic11/1
  Shift Arithmetic11/1 -> Bitwise Operator1/3
  Shift Arithmetic3/1 -> Bitwise Operator2/3
  Shift Arithmetic5/1 -> Bitwise Operator3/3
  Constant6/1 -> Shift Arithmetic5/1
  Constant5/1 -> Shift Arithmetic4/1
  R3RMdSeatOccupied_Val_read/1 -> Logical Operator/1
  Shift Arithmetic4/1 -> Bitwise Operator3/2
  Bitwise Operator3/1 -> Bitwise Operator4/1
  Bitwise Operator4/1 -> [OtherMdIsPos]
  [OtherMdIsPos] -> Bitwise Operator2/4
  [OtherMdIsPos] -> Bitwise Operator/4
  [OtherMdIsPos] -> Bitwise Operator1/4
  Data Type Conversion6/1 -> Bitwise Operator3/1
  Constant4/1 -> Shift Arithmetic6/1
  Shift Arithmetic6/1 -> Bitwise Operator3/4
  Md53IsTargetPos/1 -> Data Type Conversion7/1
  Data Type Conversion7/1 -> Shift Arithmetic7/1
  Shift Arithmetic7/1 -> Bitwise Operator2/5
  Md53IsTargetPosAlready/1 -> Data Type Conversion9/1
  Data Type Conversion9/1 -> Shift Arithmetic9/1
  Shift Arithmetic9/1 -> Bitwise Operator/5
  Constant7/1 -> Data Type Conversion10/1
  Data Type Conversion10/1 -> Shift Arithmetic10/1
  Shift Arithmetic10/1 -> Bitwise Operator1/5
  Shift Arithmetic12/1 -> Bitwise Operator2/6
  Data Type Conversion12/1 -> Shift Arithmetic12/1
  Md28IsTargetPos/1 -> Data Type Conversion12/1
  Md28IsTargetPosAlready/1 -> Data Type Conversion13/1
  Data Type Conversion13/1 -> Shift Arithmetic13/1
  Shift Arithmetic13/1 -> Bitwise Operator/6
  Shift Arithmetic14/1 -> Bitwise Operator1/6
  Data Type Conversion15/1 -> Shift Arithmetic14/1
  Md28IsTargetPosZone/1 -> Data Type Conversion15/1
  Shift Arithmetic15/1 -> Bitwise Operator3/5
  Constant8/1 -> Shift Arithmetic15/1
  Shift Arithmetic16/1 -> Bitwise Operator3/6
  Constant9/1 -> Shift Arithmetic16/1
  Md56IsTargetPos/1 -> Data Type Conversion16/1
  Data Type Conversion16/1 -> Shift Arithmetic17/1
  Shift Arithmetic17/1 -> Bitwise Operator2/7
  Shift Arithmetic18/1 -> Bitwise Operator/7
  Data Type Conversion17/1 -> Shift Arithmetic18/1
  Md56IsTargetPosAlready/1 -> Data Type Conversion17/1
  Md56IsTargetPosZone/1 -> Data Type Conversion18/1
  Data Type Conversion18/1 -> Shift Arithmetic19/1
  Shift Arithmetic19/1 -> Bitwise Operator1/7
  Constant10/1 -> Shift Arithmetic20/1
  Shift Arithmetic20/1 -> Bitwise Operator3/7
  Shift Arithmetic21/1 -> Bitwise Operator3/8
  Constant11/1 -> Shift Arithmetic21/1
  Shift Arithmetic22/1 -> Bitwise Operator2/8
  Data Type Conversion19/1 -> Shift Arithmetic22/1
  Md57IsTargetPos/1 -> Data Type Conversion19/1
  Md58IsTargetPos/1 -> Data Type Conversion20/1
  Data Type Conversion20/1 -> Shift Arithmetic23/1
  Shift Arithmetic23/1 -> Bitwise Operator2/9
  Md57IsTargetPosAlready/1 -> Data Type Conversion21/1
  Data Type Conversion21/1 -> Shift Arithmetic24/1
  Shift Arithmetic24/1 -> Bitwise Operator/8
  Shift Arithmetic25/1 -> Bitwise Operator/9
  Data Type Conversion22/1 -> Shift Arithmetic25/1
  Md58IsTargetPosAlready/1 -> Data Type Conversion22/1
  Shift Arithmetic26/1 -> Bitwise Operator1/8
  Data Type Conversion23/1 -> Shift Arithmetic26/1
  Md57IsTargetPosZone/1 -> Data Type Conversion23/1
  Md58IsTargetPosZone/1 -> Data Type Conversion24/1
  Data Type Conversion24/1 -> Shift Arithmetic27/1
  Shift Arithmetic27/1 -> Bitwise Operator1/9
  Constant12/1 -> Data Type Conversion14/1
  VIPLIsTargetPosZone/1 -> Terminator/1
  Constant13/1 -> Data Type Conversion6/1
  Logical Operator/1 -> Terminator1/1
  Constant14/1 -> Shift Arithmetic28/1
  Shift Arithmetic28/1 -> Bitwise Operator3/9
  Shift Arithmetic29/1 -> Bitwise Operator3/10
  Constant15/1 -> Shift Arithmetic29/1
  Shift Arithmetic30/1 -> Bitwise Operator2/10
  Data Type Conversion25/1 -> Shift Arithmetic30/1
  Md61IsTargetPos/1 -> Data Type Conversion25/1
  Md62IsTargetPos/1 -> Data Type Conversion26/1
  Data Type Conversion26/1 -> Shift Arithmetic31/1
  Shift Arithmetic31/1 -> Bitwise Operator2/11
  Md61IsTargetPosAlready/1 -> Data Type Conversion27/1
  Data Type Conversion27/1 -> Shift Arithmetic32/1
  Shift Arithmetic32/1 -> Bitwise Operator/10
  Shift Arithmetic33/1 -> Bitwise Operator/11
  Data Type Conversion28/1 -> Shift Arithmetic33/1
  Md62IsTargetPosAlready/1 -> Data Type Conversion28/1
  Shift Arithmetic34/1 -> Bitwise Operator1/10
  Data Type Conversion29/1 -> Shift Arithmetic34/1
  Md61IsTargetPosZone/1 -> Data Type Conversion29/1
  Md62IsTargetPosZone/1 -> Data Type Conversion30/1
  Data Type Conversion30/1 -> Shift Arithmetic35/1
  Shift Arithmetic35/1 -> Bitwise Operator1/11
  Constant16/1 -> Shift Arithmetic36/1
  Shift Arithmetic36/1 -> Bitwise Operator3/11
  Shift Arithmetic37/1 -> Bitwise Operator2/12
  Data Type Conversion31/1 -> Shift Arithmetic37/1
  Md15IsTargetPos/1 -> Data Type Conversion31/1
  Shift Arithmetic38/1 -> Bitwise Operator/12
  Data Type Conversion32/1 -> Shift Arithmetic38/1
  Md15IsTargetPosAlready/1 -> Data Type Conversion32/1
  Data Type Conversion33/1 -> Shift Arithmetic39/1
  Md15IsTargetPosZone/1 -> Data Type Conversion33/1
  Shift Arithmetic39/1 -> Bitwise Operator1/12

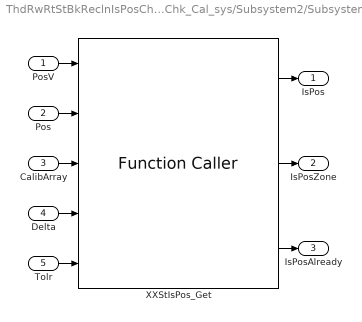
== system ThdRwRtStBkReclnIsPosChk/ThdRwRtStBkReclnIsPosChk_Cal_sys/Subsystem2/Subsystem10 ==
  PosV : Inport
  Pos : Inport  Port=2
  CalibArray : Inport  Port=3
  Delta : Inport  Port=4
  Tolr : Inport  Port=5
  XXStIsPos_Get : FunctionCaller  FunctionPrototype=[IsPos,IsPosZone,IsPosAlready] = XXStIsPos_Get(PosV,Pos,CalibArray,Delta,Tolr)  InputArgumentSpecifications=boolean(true), uint16(1), uint16([1;1;1]), uint16(1), uint16(1)  OutputArgumentSpecifications=boolean(true), boolean(true), boolean(true)
  IsPos : Outport
  IsPosZone : Outport  Port=2
  IsPosAlready : Outport  Port=3
  wires:
  PosV/1 -> XXStIsPos_Get/1
  XXStIsPos_Get/3 -> IsPosAlready/1
  Tolr/1 -> XXStIsPos_Get/5
  XXStIsPos_Get/1 -> IsPos/1
  XXStIsPos_Get/2 -> IsPosZone/1
  CalibArray/1 -> XXStIsPos_Get/3
  Delta/1 -> XXStIsPos_Get/4
  Pos/1 -> XXStIsPos_Get/2

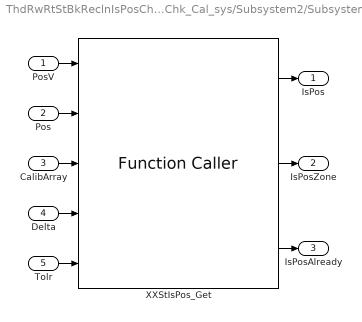
== system ThdRwRtStBkReclnIsPosChk/ThdRwRtStBkReclnIsPosChk_Cal_sys/Subsystem2/Subsystem11 ==
  PosV : Inport
  Pos : Inport  Port=2
  CalibArray : Inport  Port=3
  Delta : Inport  Port=4
  Tolr : Inport  Port=5
  XXStIsPos_Get : FunctionCaller  FunctionPrototype=[IsPos,IsPosZone,IsPosAlready] = XXStIsPos_Get(PosV,Pos,CalibArray,Delta,Tolr)  InputArgumentSpecifications=boolean(true), uint16(1), uint16([1;1;1]), uint16(1), uint16(1)  OutputArgumentSpecifications=boolean(true), boolean(true), boolean(true)
  IsPos : Outport
  IsPosZone : Outport  Port=2
  IsPosAlready : Outport  Port=3
  wires:
  Pos/1 -> XXStIsPos_Get/2
  Delta/1 -> XXStIsPos_Get/4
  CalibArray/1 -> XXStIsPos_Get/3
  XXStIsPos_Get/2 -> IsPosZone/1
  XXStIsPos_Get/1 -> IsPos/1
  Tolr/1 -> XXStIsPos_Get/5
  XXStIsPos_Get/3 -> IsPosAlready/1
  PosV/1 -> XXStIsPos_Get/1

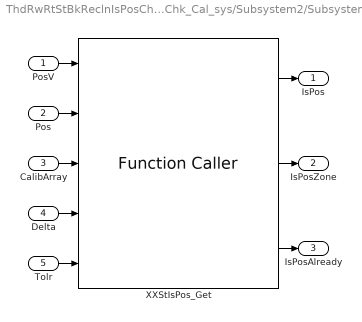
== system ThdRwRtStBkReclnIsPosChk/ThdRwRtStBkReclnIsPosChk_Cal_sys/Subsystem2/Subsystem12 ==
  PosV : Inport
  Pos : Inport  Port=2
  CalibArray : Inport  Port=3
  Delta : Inport  Port=4
  Tolr : Inport  Port=5
  XXStIsPos_Get : FunctionCaller  FunctionPrototype=[IsPos,IsPosZone,IsPosAlready] = XXStIsPos_Get(PosV,Pos,CalibArray,Delta,Tolr)  InputArgumentSpecifications=boolean(true), uint16(1), uint16([1;1;1]), uint16(1), uint16(1)  OutputArgumentSpecifications=boolean(true), boolean(true), boolean(true)
  IsPos : Outport
  IsPosZone : Outport  Port=2
  IsPosAlready : Outport  Port=3
  wires:
  Pos/1 -> XXStIsPos_Get/2
  Delta/1 -> XXStIsPos_Get/4
  CalibArray/1 -> XXStIsPos_Get/3
  XXStIsPos_Get/2 -> IsPosZone/1
  XXStIsPos_Get/1 -> IsPos/1
  Tolr/1 -> XXStIsPos_Get/5
  XXStIsPos_Get/3 -> IsPosAlready/1
  PosV/1 -> XXStIsPos_Get/1

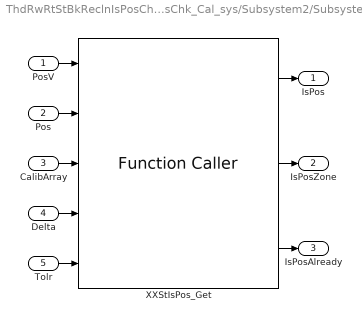
== system ThdRwRtStBkReclnIsPosChk/ThdRwRtStBkReclnIsPosChk_Cal_sys/Subsystem2/Subsystem2 ==
  PosV : Inport
  Pos : Inport  Port=2
  CalibArray : Inport  Port=3
  Delta : Inport  Port=4
  Tolr : Inport  Port=5
  XXStIsPos_Get : FunctionCaller  FunctionPrototype=[IsPos,IsPosZone,IsPosAlready] = XXStIsPos_Get(PosV,Pos,CalibArray,Delta,Tolr)  InputArgumentSpecifications=boolean(true), uint16(1), uint16([1;1;1]), uint16(1), uint16(1)  OutputArgumentSpecifications=boolean(true), boolean(true), boolean(true)
  IsPos : Outport
  IsPosZone : Outport  Port=2
  IsPosAlready : Outport  Port=3
  wires:
  PosV/1 -> XXStIsPos_Get/1
  XXStIsPos_Get/3 -> IsPosAlready/1
  Tolr/1 -> XXStIsPos_Get/5
  XXStIsPos_Get/1 -> IsPos/1
  XXStIsPos_Get/2 -> IsPosZone/1
  CalibArray/1 -> XXStIsPos_Get/3
  Delta/1 -> XXStIsPos_Get/4
  Pos/1 -> XXStIsPos_Get/2

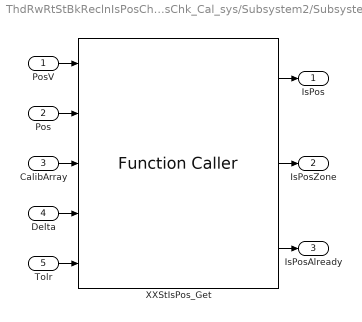
== system ThdRwRtStBkReclnIsPosChk/ThdRwRtStBkReclnIsPosChk_Cal_sys/Subsystem2/Subsystem3 ==
  PosV : Inport
  Pos : Inport  Port=2
  CalibArray : Inport  Port=3
  Delta : Inport  Port=4
  Tolr : Inport  Port=5
  XXStIsPos_Get : FunctionCaller  FunctionPrototype=[IsPos,IsPosZone,IsPosAlready] = XXStIsPos_Get(PosV,Pos,CalibArray,Delta,Tolr)  InputArgumentSpecifications=boolean(true), uint16(1), uint16([1;1;1]), uint16(1), uint16(1)  OutputArgumentSpecifications=boolean(true), boolean(true), boolean(true)
  IsPos : Outport
  IsPosZone : Outport  Port=2
  IsPosAlready : Outport  Port=3
  wires:
  PosV/1 -> XXStIsPos_Get/1
  XXStIsPos_Get/3 -> IsPosAlready/1
  Tolr/1 -> XXStIsPos_Get/5
  XXStIsPos_Get/1 -> IsPos/1
  XXStIsPos_Get/2 -> IsPosZone/1
  CalibArray/1 -> XXStIsPos_Get/3
  Delta/1 -> XXStIsPos_Get/4
  Pos/1 -> XXStIsPos_Get/2

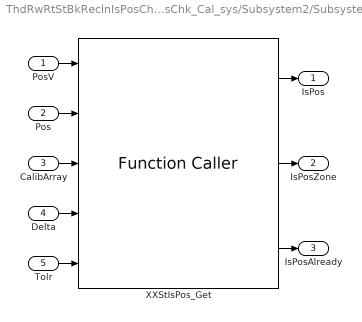
== system ThdRwRtStBkReclnIsPosChk/ThdRwRtStBkReclnIsPosChk_Cal_sys/Subsystem2/Subsystem4 ==
  PosV : Inport
  Pos : Inport  Port=2
  CalibArray : Inport  Port=3
  Delta : Inport  Port=4
  Tolr : Inport  Port=5
  XXStIsPos_Get : FunctionCaller  FunctionPrototype=[IsPos,IsPosZone,IsPosAlready] = XXStIsPos_Get(PosV,Pos,CalibArray,Delta,Tolr)  InputArgumentSpecifications=boolean(true), uint16(1), uint16([1;1;1]), uint16(1), uint16(1)  OutputArgumentSpecifications=boolean(true), boolean(true), boolean(true)
  IsPos : Outport
  IsPosZone : Outport  Port=2
  IsPosAlready : Outport  Port=3
  wires:
  PosV/1 -> XXStIsPos_Get/1
  XXStIsPos_Get/3 -> IsPosAlready/1
  Tolr/1 -> XXStIsPos_Get/5
  XXStIsPos_Get/1 -> IsPos/1
  XXStIsPos_Get/2 -> IsPosZone/1
  CalibArray/1 -> XXStIsPos_Get/3
  Delta/1 -> XXStIsPos_Get/4
  Pos/1 -> XXStIsPos_Get/2

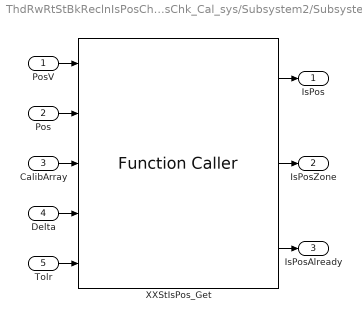
== system ThdRwRtStBkReclnIsPosChk/ThdRwRtStBkReclnIsPosChk_Cal_sys/Subsystem2/Subsystem5 ==
  PosV : Inport
  Pos : Inport  Port=2
  CalibArray : Inport  Port=3
  Delta : Inport  Port=4
  Tolr : Inport  Port=5
  XXStIsPos_Get : FunctionCaller  FunctionPrototype=[IsPos,IsPosZone,IsPosAlready] = XXStIsPos_Get(PosV,Pos,CalibArray,Delta,Tolr)  InputArgumentSpecifications=boolean(true), uint16(1), uint16([1;1;1]), uint16(1), uint16(1)  OutputArgumentSpecifications=boolean(true), boolean(true), boolean(true)
  IsPos : Outport
  IsPosZone : Outport  Port=2
  IsPosAlready : Outport  Port=3
  wires:
  Pos/1 -> XXStIsPos_Get/2
  Delta/1 -> XXStIsPos_Get/4
  CalibArray/1 -> XXStIsPos_Get/3
  XXStIsPos_Get/2 -> IsPosZone/1
  XXStIsPos_Get/1 -> IsPos/1
  Tolr/1 -> XXStIsPos_Get/5
  XXStIsPos_Get/3 -> IsPosAlready/1
  PosV/1 -> XXStIsPos_Get/1

== system ThdRwRtStBkReclnIsPosChk/ThdRwRtStBkReclnIsPosChk_Cal_sys/Subsystem2/Subsystem6 ==
  PosV : Inport
  Pos : Inport  Port=2
  CalibArray : Inport  Port=3
  Delta : Inport  Port=4
  Tolr : Inport  Port=5
  XXStIsPos_Get : FunctionCaller  FunctionPrototype=[IsPos,IsPosZone,IsPosAlready] = XXStIsPos_Get(PosV,Pos,CalibArray,Delta,Tolr)  InputArgumentSpecifications=boolean(true), uint16(1), uint16([1;1;1]), uint16(1), uint16(1)  OutputArgumentSpecifications=boolean(true), boolean(true), boolean(true)
  IsPos : Outport
  IsPosZone : Outport  Port=2
  IsPosAlready : Outport  Port=3
  wires:
  PosV/1 -> XXStIsPos_Get/1
  XXStIsPos_Get/3 -> IsPosAlready/1
  Tolr/1 -> XXStIsPos_Get/5
  XXStIsPos_Get/1 -> IsPos/1
  XXStIsPos_Get/2 -> IsPosZone/1
  CalibArray/1 -> XXStIsPos_Get/3
  Delta/1 -> XXStIsPos_Get/4
  Pos/1 -> XXStIsPos_Get/2

== system ThdRwRtStBkReclnIsPosChk/ThdRwRtStBkReclnIsPosChk_Cal_sys/Subsystem2/Subsystem7 ==
  PosV : Inport
  Pos : Inport  Port=2
  CalibArray : Inport  Port=3
  Delta : Inport  Port=4
  Tolr : Inport  Port=5
  XXStIsPos_Get : FunctionCaller  FunctionPrototype=[IsPos,IsPosZone,IsPosAlready] = XXStIsPos_Get(PosV,Pos,CalibArray,Delta,Tolr)  InputArgumentSpecifications=boolean(true), uint16(1), uint16([1;1;1]), uint16(1), uint16(1)  OutputArgumentSpecifications=boolean(true), boolean(true), boolean(true)
  IsPos : Outport
  IsPosZone : Outport  Port=2
  IsPosAlready : Outport  Port=3
  wires:
  Pos/1 -> XXStIsPos_Get/2
  Delta/1 -> XXStIsPos_Get/4
  CalibArray/1 -> XXStIsPos_Get/3
  XXStIsPos_Get/2 -> IsPosZone/1
  XXStIsPos_Get/1 -> IsPos/1
  Tolr/1 -> XXStIsPos_Get/5
  XXStIsPos_Get/3 -> IsPosAlready/1
  PosV/1 -> XXStIsPos_Get/1

== system ThdRwRtStBkReclnIsPosChk/ThdRwRtStBkReclnIsPosChk_Cal_sys/Subsystem2/Subsystem8 ==
  PosV : Inport
  Pos : Inport  Port=2
  CalibArray : Inport  Port=3
  Delta : Inport  Port=4
  Tolr : Inport  Port=5
  XXStIsPos_Get : FunctionCaller  FunctionPrototype=[IsPos,IsPosZone,IsPosAlready] = XXStIsPos_Get(PosV,Pos,CalibArray,Delta,Tolr)  InputArgumentSpecifications=boolean(true), uint16(1), uint16([1;1;1]), uint16(1), uint16(1)  OutputArgumentSpecifications=boolean(true), boolean(true), boolean(true)
  IsPos : Outport
  IsPosZone : Outport  Port=2
  IsPosAlready : Outport  Port=3
  wires:
  PosV/1 -> XXStIsPos_Get/1
  XXStIsPos_Get/3 -> IsPosAlready/1
  Tolr/1 -> XXStIsPos_Get/5
  XXStIsPos_Get/1 -> IsPos/1
  XXStIsPos_Get/2 -> IsPosZone/1
  CalibArray/1 -> XXStIsPos_Get/3
  Delta/1 -> XXStIsPos_Get/4
  Pos/1 -> XXStIsPos_Get/2

== system ThdRwRtStBkReclnIsPosChk/ThdRwRtStBkReclnIsPosChk_Cal_sys/Subsystem2/Subsystem9 ==
  PosV : Inport
  Pos : Inport  Port=2
  CalibArray : Inport  Port=3
  Delta : Inport  Port=4
  Tolr : Inport  Port=5
  XXStIsPos_Get : FunctionCaller  FunctionPrototype=[IsPos,IsPosZone,IsPosAlready] = XXStIsPos_Get(PosV,Pos,CalibArray,Delta,Tolr)  InputArgumentSpecifications=boolean(true), uint16(1), uint16([1;1;1]), uint16(1), uint16(1)  OutputArgumentSpecifications=boolean(true), boolean(true), boolean(true)
  IsPos : Outport
  IsPosZone : Outport  Port=2
  IsPosAlready : Outport  Port=3
  wires:
  Pos/1 -> XXStIsPos_Get/2
  Delta/1 -> XXStIsPos_Get/4
  CalibArray/1 -> XXStIsPos_Get/3
  XXStIsPos_Get/2 -> IsPosZone/1
  XXStIsPos_Get/1 -> IsPos/1
  Tolr/1 -> XXStIsPos_Get/5
  XXStIsPos_Get/3 -> IsPosAlready/1
  PosV/1 -> XXStIsPos_Get/1
